simulink model "arduino_output_test"  (R2021a)
settings: Solver=VariableStepAuto  StartTime=0.0  StopTime=10.0  RelTol=1e-3
libraries: arduinolib x4
settings Model: Creator=Intuito_PC  LastModifiedBy=Intuito_PC

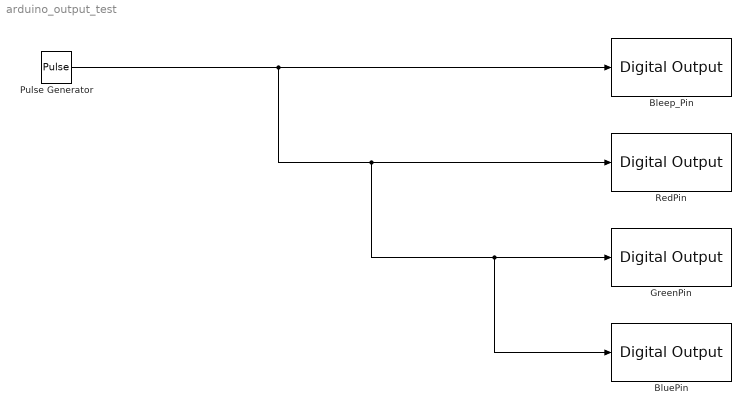
== system arduino_output_test ==
  Bleep_Pin : arduinolib/Digital Output  pinNumber=5  Direction=output  blockPlatform=arduino
  BluePin : arduinolib/Digital Output  pinNumber=5  Direction=output  blockPlatform=arduino
  GreenPin : arduinolib/Digital Output  pinNumber=5  Direction=output  blockPlatform=arduino
  Pulse Generator : DiscretePulseGenerator  PulseType=Time based  Period=1  PulseWidth=5
  RedPin : arduinolib/Digital Output  pinNumber=5  Direction=output  blockPlatform=arduino
  wires:
  Pulse Generator/1 -> BluePin/1, GreenPin/1, RedPin/1, Bleep_Pin/1
